simulink model "motor_identifica"  (R2024b)
settings: Solver=VariableStepAuto  StartTime=0.0  StopTime=10.0  RelTol=1e-3
undefined symbols (not defined in the file or in its folder): A, B
settings Model: Creator=cagla  LastModifiedBy=cagla

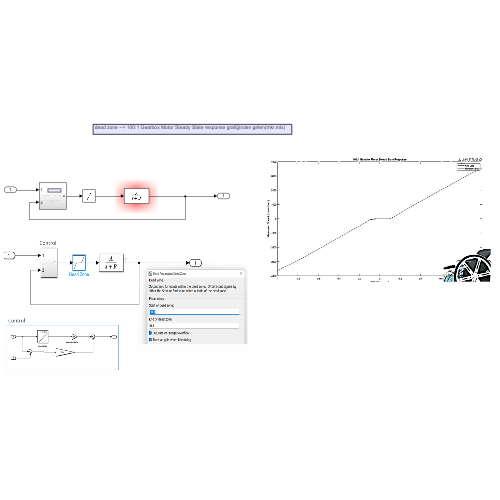
[thumbnail: Simulink's stored preview of the top-level diagram]
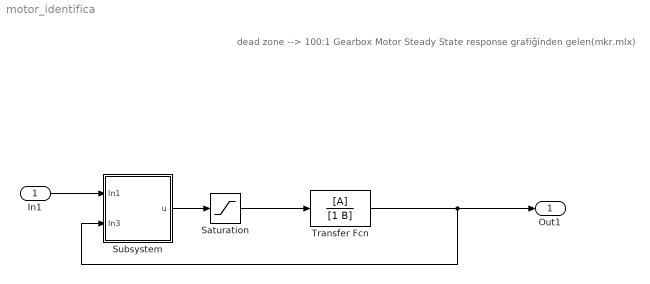
== system motor_identifica ==
  note: dead zone --> 100:1 Gearbox Motor Steady State response grafiğinden gelen(mkr.mlx)
  In1 : Inport
  Saturation : Saturate
  Subsystem : Subsystem
  Transfer Fcn : TransferFcn  Numerator=[A]  Denominator=[1 B]
  Out1 : Outport
  wires:
  Saturation/1 -> Transfer Fcn/1
  Transfer Fcn/1 -> Subsystem/2(In3), Out1/1
  In1/1 -> Subsystem/1(In1)
  Subsystem/1(u) -> Saturation/1

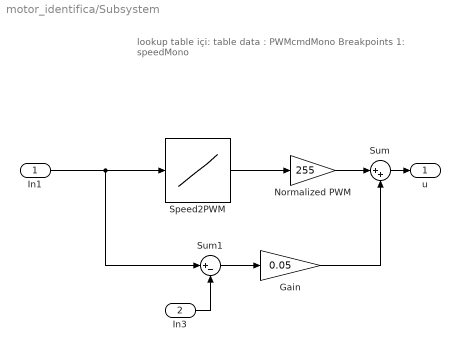
== system motor_identifica/Subsystem ==
  note: lookup table içi:
      | table data : PWMcmdMono
      | Breakpoints 1: speedMono
  In1 : Inport
  In3 : Inport  Port=2
  Gain : Gain  Gain=0.05
  Normalized PWM : Gain  Gain=255
  Speed2PWM : Lookup_n-D  NumberOfTableDimensions=1  BreakpointsForDimension1=[-5:5]  Table=tanh([-5:5])  InternalRulePriority=Speed  RndMeth=Simplest
  Sum : Sum  Inputs=|++
  Sum1 : Sum  Inputs=|+-
  u : Outport
  wires:
  Speed2PWM/1 -> Normalized PWM/1
  Sum/1 -> u/1
  In1/1 -> Sum1/1, Speed2PWM/1
  Sum1/1 -> Gain/1
  Gain/1 -> Sum/2
  In3/1 -> Sum1/2
  Normalized PWM/1 -> Sum/1
